simulink model "PV_Module"  (R2020a)
settings: Solver=VariableStepAuto  StartTime=0.0  StopTime=4  RelTol=1e-10
values from neighbouring files (symbols this model uses):
  Eg = 1.1    [data.m]
  Isc = 8.21    [data.m]
  k = 1.38*((10)^-23)    (= 1.38e-23)    [data.m]
  ki = 0.0032    [data.m]
  n = 1.3    [data.m]
  Ns = 54    [data.m]
  q = 1.6*((10)^-19)    (= 1.6e-19)    [data.m]
  Rs = 0.221    [data.m]
  Rsh = 415.405    [data.m]
  Tn = 298    [data.m]
  Voc = 32.9    [data.m]
libraries: simulink x4, powerlib x3, re_lib x1
settings Model: Creator=Khojasteh Mirza  LastModifiedBy=Khojasteh Mirza
settings SolverCC: AlgebraicLoopSolver=LineSearch

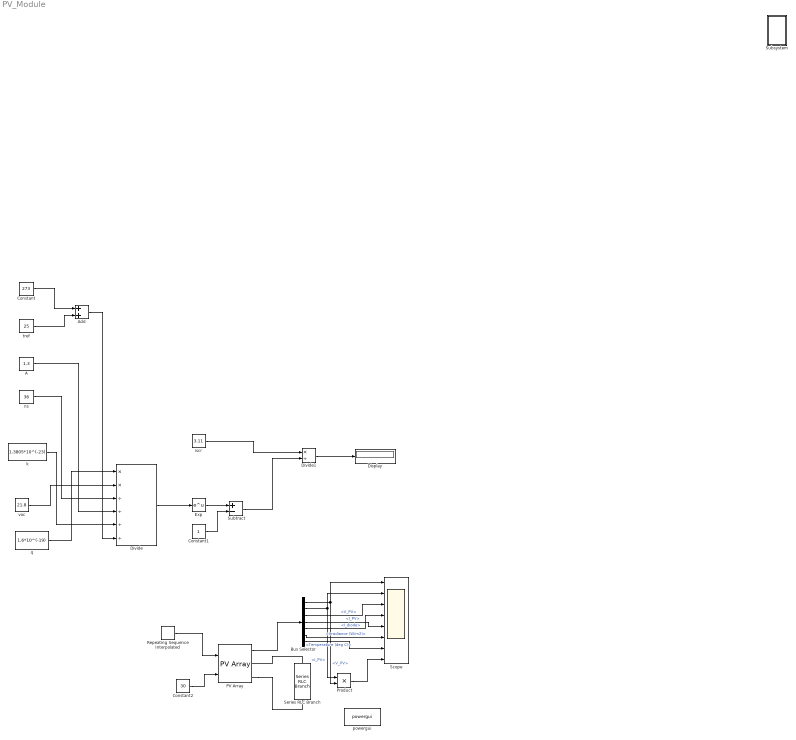
== system PV_Module ==
  A : Constant  Value=1.3
  Add : Sum
  Bus Selector : BusSelector  OutputSignals=V_PV,I_PV,V_PV,I_PV,I_diode,Irradiance (W/m2),Temperature (deg C)
  Constant : Constant  Value=273
  Constant1 : Constant
  Constant2 : Constant  Value=30
  Display : Display
  Divide : Product  Inputs=**////
  Divide1 : Product  Inputs=*/
  Exp : Math  SaturateOnIntegerOverflow=on
  PV Array : re_lib/Solar/PV Array  Npar=40  Nser=10  PlotType=array @ 1000 W/m2 & specified temperatures  S_vec="[ 1000  500  100 ]"  Temp_C_vec="[ 45 25  ]"  ModuleName=1Soltech 1STH-215-P  PlotWhenSelected=off  Pm=213.15  Ncell=60  Voc=36.3  Isc=7.84  Vm=29  Im=7.35  beta_Voc_pc=-0.36099  alpha_Isc_pc=0.102  beta_Voc=-0.13104  alpha_Isc=0.007997  IL=7.8649  I0=2.9259e-10  nI=0.98117  Rsh=313.3991  Rs=0.39383  RobustModel=off  RobustCellTemperature=25  BAL=on  Tc=1e-6  Tfilter=5e-5
  Product : Product
  Repeating Sequence Interpolated : simulink/Sources/Repeating Sequence Interpolated  OutValues=[3 1 4 2 1].'  TimeValues=[0 0.1 0.5 0.6 1].'  LookUpMeth=Interpolation-Use End Values  tsamp=0.01  OutMin=[]  OutMax=[]  OutDataTypeStr=double  OutputDataTypeScalingMode=double  OutDataType=fixdt(0,8)  OutScaling=2^-10
  Scope : Scope  NumInputPorts=8
  Series RLC Branch : powerlib/Elements/Series RLC Branch  LConnTagsString=__new0  RConnTagsString=__new0  BranchType=R  Resistance=40  Inductance=1e-3  SetiL0=off  InitialCurrent=0  Capacitance=1e-6  Setx0=off  InitialVoltage=0  Measurements=None
  Subsystem : Subsystem
  Subtract : Sum  Inputs=+-
  iscr : Constant  Value=3.11
  k : Constant  Value=1.3805*10^(-23)
  ns : Constant  Value=36
  powergui : powerlib/powergui  Priority=1  SimulationMode=Continuous  SampleTime=50e-6  frequency=60  Iterations=50  frequencyindice=0  Pbase=100e6  ErrMax=1e-4  UnitsV=kV  UnitsW=MW  buscounter=0  FunctionMessages=off  echomessages=off  EnableUseOfTLC=off  CurrentSourceSwitches=off  DisableSnubberDevices=off  DisableRonSwitches=off  DisableVfSwitches=off  DisplayEquations=off  AutomaticDiscreteSolvers=off  SolverType=Tustin/Backward Euler (TBE)  Interpol=off  ExternalGateDelay=off  methode=off  Ts=100  x0status=blocks  SPID=on  SwTol=0  HookPort=off  NonlinearTolerance=1e-4  nMaxIteration=100  ContinueOnMaxIteration=off  RestoreLinks=warning  ResistiveCurrentMeasurement=off  Frange=[0:2:500]  Ylog=off  Xlog=on  ShowGrid=off  save=off  variable=ZData  structure=0  ZoomFFT=off  StartTime=0.0  cycles=1  DisplayStyle=1  fundamental=60  FreqAxis=off  MaxFrequency=1000  frequencyindicesteady=1  RmsSteady=1  display=off
  q : Constant  Value=1.6*10^(-19)
  tref : Constant  Value=25
  voc : Constant  Value=21.8
  wires:
  Constant/1 -> Add/1
  tref/1 -> Add/2
  q/1 -> Divide/1
  voc/1 -> Divide/2
  A/1 -> Divide/4
  ns/1 -> Divide/3
  k/1 -> Divide/5
  Add/1 -> Divide/6
  Divide/1 -> Exp/1
  Exp/1 -> Subtract/1
  Constant1/1 -> Subtract/2
  iscr/1 -> Divide1/1
  Subtract/1 -> Divide1/2
  Divide1/1 -> Display/1
  Repeating Sequence Interpolated/1 -> PV Array/1
  Constant2/1 -> PV Array/2
  PV Array/1 -> Bus Selector/1
  Bus Selector/1 -> Product/2, Scope/1  "<V_PV>"
  Bus Selector/2 -> Product/1, Scope/2  "<I_PV>"
  Product/1 -> Scope/8
  Bus Selector/4 -> Scope/5  "<I_PV>"
  Bus Selector/3 -> Scope/3  "<V_PV>"
  Bus Selector/6 -> Scope/6  "<Irradiance (W/m2)>"
  Bus Selector/7 -> Scope/7  "<Temperature (deg C)>"
  Bus Selector/5 -> Scope/4  "<I_diode>"
  connections:
  Series RLC Branch/LConn1 -- PV Array/RConn1
  PV Array/RConn2 -- Series RLC Branch/RConn1

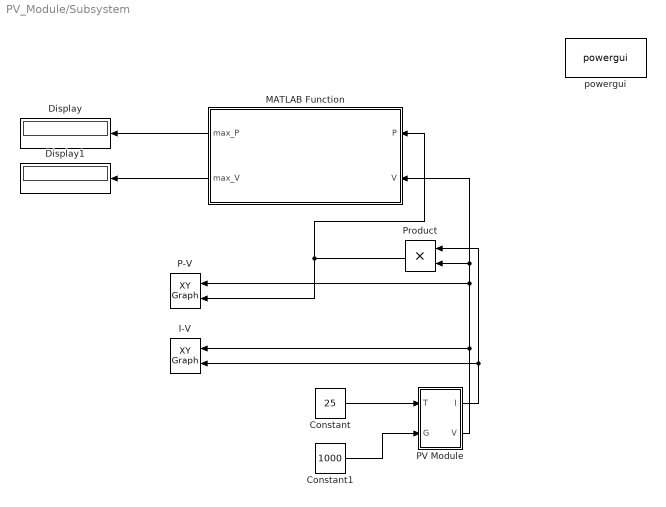
== system PV_Module/Subsystem ==
  Constant : Constant  Value=25
  Constant1 : Constant  Value=1000
  Display : Display
  Display1 : Display
  I-V : simulink/Sinks/XY Graph  xmin=0  xmax=50  ymin=0  ymax=10  st=-1
  MATLAB Function : MATLAB Function  TreatAsAtomicUnit=on
  P-V : simulink/Sinks/XY Graph  xmin=0  xmax=35  ymin=0  ymax=300  st=-1
  PV Module : Subsystem
  Product : Product
  powergui : powerlib/powergui  Priority=1  SimulationMode=Continuous  SampleTime=50e-6  frequency=60  Iterations=50  frequencyindice=60  Pbase=100e6  ErrMax=1e-4  UnitsV=kV  UnitsW=MW  buscounter=0  FunctionMessages=off  echomessages=off  EnableUseOfTLC=off  CurrentSourceSwitches=off  DisableSnubberDevices=off  DisableRonSwitches=off  DisableVfSwitches=off  DisplayEquations=off  AutomaticDiscreteSolvers=off  SolverType=Tustin/Backward Euler (TBE)  Interpol=off  ExternalGateDelay=off  methode=off  Ts=100  x0status=blocks  SPID=on  SwTol=0  HookPort=off  NonlinearTolerance=1e-4  nMaxIteration=100  ContinueOnMaxIteration=off  RestoreLinks=warning  ResistiveCurrentMeasurement=off  Frange=[0:2:500]  Ylog=off  Xlog=on  ShowGrid=off  save=off  variable=ZData  structure=0  ZoomFFT=off  StartTime=0.0  cycles=1  DisplayStyle=1  fundamental=60  FreqAxis=off  MaxFrequency=1000  frequencyindicesteady=1  RmsSteady=1  display=off
  wires:
  Constant/1 -> PV Module/1(T)
  Constant1/1 -> PV Module/2(G)
  PV Module/1(I) -> I-V/2, Product/1
  PV Module/2(V) -> Product/2, MATLAB Function/2(V), P-V/1, I-V/1
  Product/1 -> MATLAB Function/1(P), P-V/2
  MATLAB Function/1(max_P) -> Display/1
  MATLAB Function/2(max_V) -> Display1/1

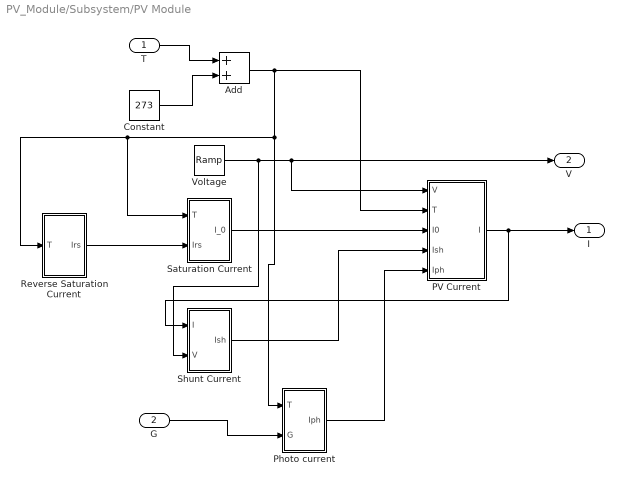
== system PV_Module/Subsystem/PV Module ==
  T : Inport
  G : Inport  Port=2
  Add : Sum
  Constant : Constant  Value=273
  PV Current : Subsystem
  Photo current : Subsystem
  Reverse Saturation Current : Subsystem
  Saturation Current : Subsystem
  Shunt Current : Subsystem
  Voltage : simulink/Sources/Ramp  slope=100  start=0  InitialOutput=0
  I : Outport
  V : Outport  Port=2
  wires:
  Shunt Current/1(Ish) -> PV Current/4(Ish)
  Voltage/1 -> Shunt Current/2(V), V/1, PV Current/1(V)
  Reverse Saturation Current/1(Irs) -> Saturation Current/2(Irs)
  Saturation Current/1(I_0) -> PV Current/3(I0)
  Constant/1 -> Add/2
  G/1 -> Photo current/2(G)
  T/1 -> Add/1
  PV Current/1(I) -> I/1, Shunt Current/1(I)
  Photo current/1(Iph) -> PV Current/5(Iph)
  Add/1 -> Saturation Current/1(T), Reverse Saturation Current/1(T), Photo current/1(T), PV Current/2(T)

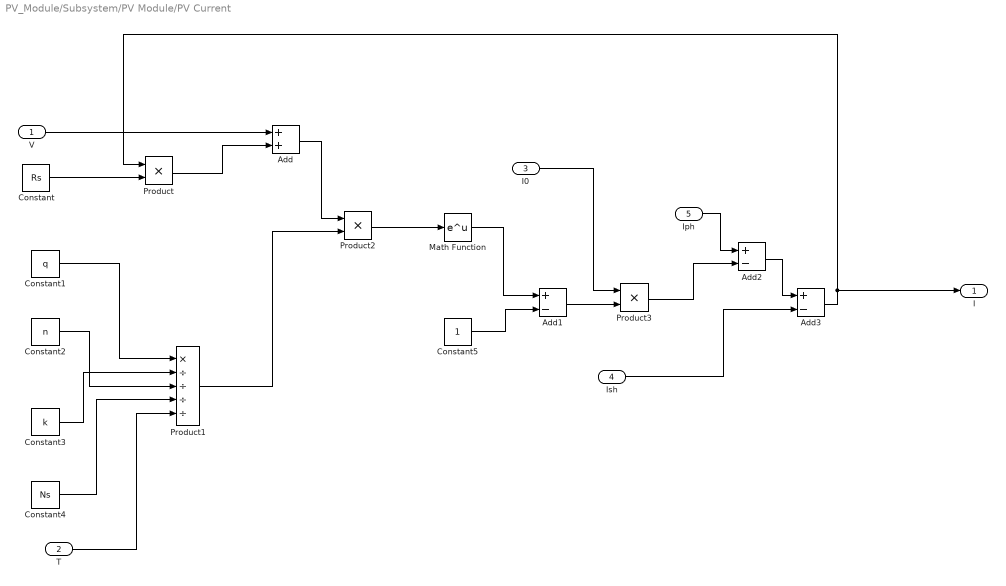
== system PV_Module/Subsystem/PV Module/PV Current ==
  V : Inport
  T : Inport  Port=2
  I0 : Inport  Port=3
  Ish : Inport  Port=4
  Iph : Inport  Port=5
  Add : Sum
  Add1 : Sum  Inputs=+-
  Add2 : Sum  Inputs=+-
  Add3 : Sum  Inputs=+-
  Constant : Constant  Value=Rs
  Constant1 : Constant  Value=q
  Constant2 : Constant  Value=n
  Constant3 : Constant  Value=k
  Constant4 : Constant  Value=Ns
  Constant5 : Constant
  Math Function : Math  SaturateOnIntegerOverflow=on
  Product : Product
  Product1 : Product  Inputs=*////
  Product2 : Product
  Product3 : Product
  I : Outport
  wires:
  Constant3/1 -> Product1/2
  Constant/1 -> Product/2
  Math Function/1 -> Add1/1
  Iph/1 -> Add2/1
  Product2/1 -> Math Function/1
  I0/1 -> Product3/1
  Ish/1 -> Add3/2
  Product/1 -> Add/2
  Constant4/1 -> Product1/4
  Add/1 -> Product2/1
  Add3/1 -> I/1, Product/1
  Add1/1 -> Product3/2
  Constant2/1 -> Product1/3
  Add2/1 -> Add3/1
  T/1 -> Product1/5
  Product3/1 -> Add2/2
  V/1 -> Add/1
  Constant1/1 -> Product1/1
  Constant5/1 -> Add1/2
  Product1/1 -> Product2/2

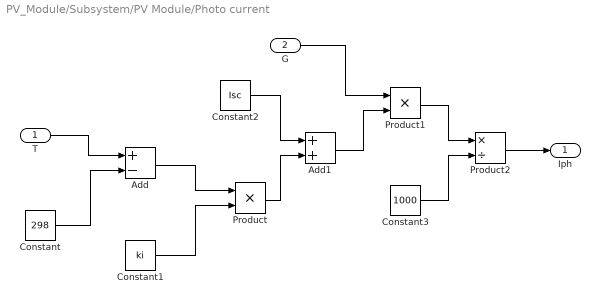
== system PV_Module/Subsystem/PV Module/Photo current ==
  T : Inport
  G : Inport  Port=2
  Add : Sum  Inputs=+-
  Add1 : Sum
  Constant : Constant  Value=298
  Constant1 : Constant  Value=ki
  Constant2 : Constant  Value=Isc
  Constant3 : Constant  Value=1000
  Product : Product
  Product1 : Product
  Product2 : Product  Inputs=*/
  Iph : Outport
  wires:
  Add/1 -> Product/1
  T/1 -> Add/1
  Constant2/1 -> Add1/1
  Constant/1 -> Add/2
  Product/1 -> Add1/2
  Constant1/1 -> Product/2
  G/1 -> Product1/1
  Constant3/1 -> Product2/2
  Add1/1 -> Product1/2
  Product1/1 -> Product2/1
  Product2/1 -> Iph/1

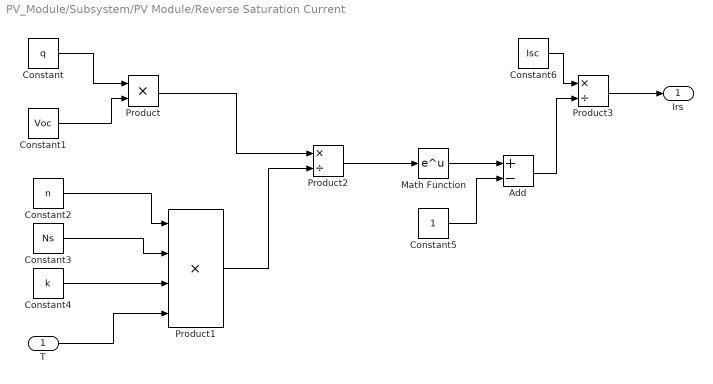
== system PV_Module/Subsystem/PV Module/Reverse Saturation Current ==
  T : Inport
  Add : Sum  Inputs=+-
  Constant : Constant  Value=q
  Constant1 : Constant  Value=Voc
  Constant2 : Constant  Value=n
  Constant3 : Constant  Value=Ns
  Constant4 : Constant  Value=k
  Constant5 : Constant
  Constant6 : Constant  Value=Isc
  Math Function : Math  SaturateOnIntegerOverflow=on
  Product : Product
  Product1 : Product  Inputs=4
  Product2 : Product  Inputs=*/
  Product3 : Product  Inputs=*/
  Irs : Outport
  wires:
  Constant6/1 -> Product3/1
  Add/1 -> Product3/2
  Constant5/1 -> Add/2
  Constant3/1 -> Product1/2
  Product3/1 -> Irs/1
  Product1/1 -> Product2/2
  Math Function/1 -> Add/1
  Product/1 -> Product2/1
  Constant2/1 -> Product1/1
  Product2/1 -> Math Function/1
  Constant/1 -> Product/1
  Constant1/1 -> Product/2
  T/1 -> Product1/4
  Constant4/1 -> Product1/3

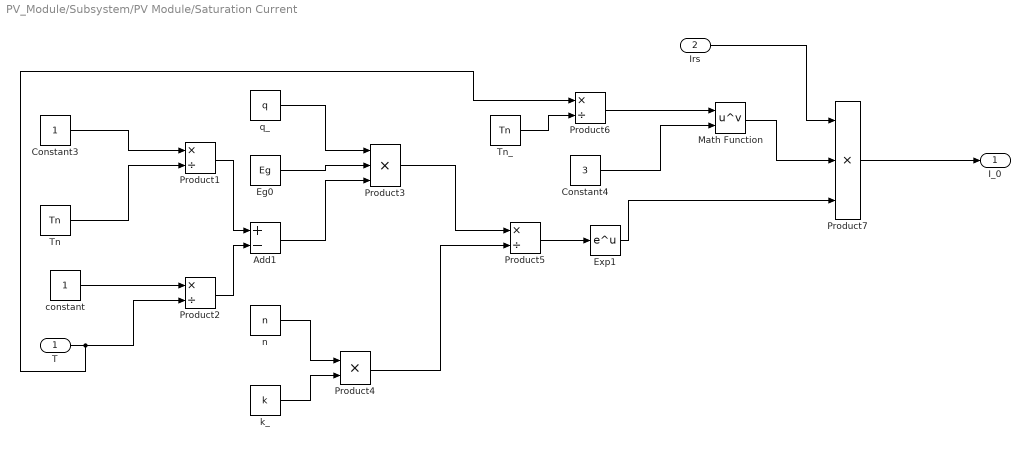
== system PV_Module/Subsystem/PV Module/Saturation Current ==
  T : Inport
  Irs : Inport  Port=2
  Add1 : Sum  Inputs=+-
  Constant3 : Constant
  Constant4 : Constant  Value=3
  Eg0 : Constant  Value=Eg
  Exp1 : Math  SaturateOnIntegerOverflow=on
  Math Function : Math  Operator=pow  SaturateOnIntegerOverflow=on
  Product{1..2,5..6} (4 alike) : Product  Inputs=*/
  Product3 : Product  Inputs=***
  Product4 : Product  Inputs=**
  Product7 : Product  Inputs=3
  Tn : Constant  Value=Tn
  Tn_ : Constant  Value=Tn
  constant : Constant
  k_ : Constant  Value=k
  n : Constant  Value=n
  q_ : Constant  Value=q
  I_0 : Outport
  wires:
  T/1 -> Product2/2, Product6/1
  Product1/1 -> Add1/1
  constant/1 -> Product2/1
  Irs/1 -> Product7/1
  Tn_/1 -> Product6/2
  Product5/1 -> Exp1/1
  Product3/1 -> Product5/1
  q_/1 -> Product3/1
  Exp1/1 -> Product7/3
  Product2/1 -> Add1/2
  Product4/1 -> Product5/2
  Constant4/1 -> Math Function/2
  Math Function/1 -> Product7/2
  Tn/1 -> Product1/2
  Product6/1 -> Math Function/1
  k_/1 -> Product4/2
  Constant3/1 -> Product1/1
  Eg0/1 -> Product3/2
  n/1 -> Product4/1
  Add1/1 -> Product3/3
  Product7/1 -> I_0/1

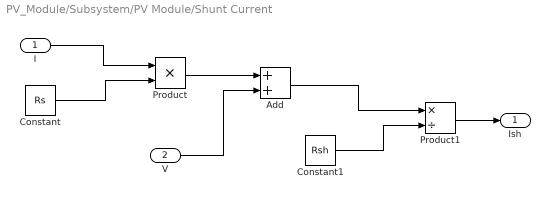
== system PV_Module/Subsystem/PV Module/Shunt Current ==
  I : Inport
  V : Inport  Port=2
  Add : Sum
  Constant : Constant  Value=Rs
  Constant1 : Constant  Value=Rsh
  Product : Product
  Product1 : Product  Inputs=*/
  Ish : Outport
  wires:
  Product1/1 -> Ish/1
  Constant/1 -> Product/2
  Constant1/1 -> Product1/2
  V/1 -> Add/2
  Product/1 -> Add/1
  Add/1 -> Product1/1
  I/1 -> Product/1

== matlab function PV_Module/Subsystem/MATLAB Function ==
  settings: updateMethod=DISCRETE
  data: P input; max_P output; V input; max_V output
function [max_P, max_V] = max_val(P,V)

persistent Ppre Vpre

if isempty(Ppre)
    Ppre = 0;
    Vpre = 0;
end

if (Ppre > P)
    max_P    = Ppre;
    max_V = Vpre;
    
else
    max_P    = P;
    max_V = V;
end
Ppre = max_P;
Vpre = max_V;
